simulink model "MPCPF_kinematics"  (R2016a)
settings: Solver=ode4  StartTime=0.0  StopTime=300  FixedStep=Ts  RelTol=1e-3
values from neighbouring files (symbols this model uses):
  Ts = 0.1    [CPFMPC_Lyapunovbased.mat]    (also in CPFMPC_NoTerminalConstraint.mat; Coordination.m; Data_StrategyII_No_Constraint.mat; Data_StrategyI_Constraint.mat = 0.2)
settings Model: Creator=hung  LastModifiedBy=hung

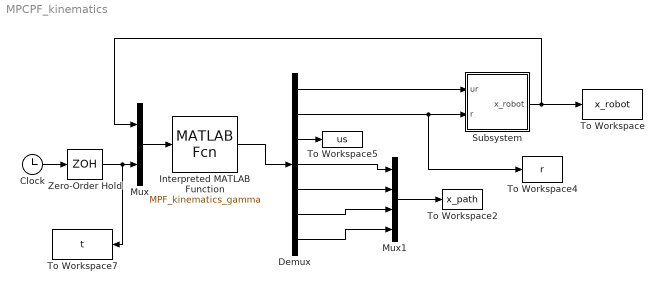
== system MPCPF_kinematics ==
  Clock : Clock
  Demux : Demux  Outputs=7
  Interpreted MATLAB Function : MATLABFcn  MATLABFcn=MPF_kinematics_gamma  OutputDimensions=7
  Mux : Mux  Inputs=2
  Mux1 : Mux
  Subsystem : Subsystem
  To Workspace : ToWorkspace  VariableName=x_robot  SampleTime=-1
  To Workspace2 : ToWorkspace  VariableName=x_path  SampleTime=-1
  To Workspace4 : ToWorkspace  VariableName=r  SampleTime=-1
  To Workspace5 : ToWorkspace  VariableName=us  SampleTime=-1
  To Workspace7 : ToWorkspace  VariableName=t  SampleTime=Ts
  Zero-Order Hold : ZeroOrderHold  SampleTime=Ts
  wires:
  Interpreted MATLAB Function/1 -> Demux/1
  Mux/1 -> Interpreted MATLAB Function/1
  Clock/1 -> Zero-Order Hold/1
  Zero-Order Hold/1 -> Mux/2, To Workspace7/1
  Demux/2 -> To Workspace4/1, Subsystem/2(r)
  Demux/4 -> Mux1/1
  Demux/5 -> Mux1/2
  Mux1/1 -> To Workspace2/1
  Demux/3 -> To Workspace5/1
  Demux/6 -> Mux1/3
  Demux/7 -> Mux1/4
  Demux/1 -> Subsystem/1(ur)
  Subsystem/1(x_robot) -> Mux/1, To Workspace/1

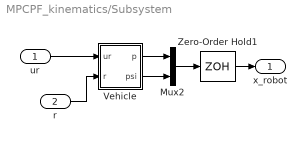
== system MPCPF_kinematics/Subsystem ==
  ur : Inport
  r : Inport  Port=2
  Mux2 : Mux  Inputs=2
  Vehicle : Subsystem
  Zero-Order Hold1 : ZeroOrderHold  SampleTime=Ts
  x_robot : Outport
  wires:
  Vehicle/2(psi) -> Mux2/2
  Mux2/1 -> Zero-Order Hold1/1
  r/1 -> Vehicle/2(r)
  Zero-Order Hold1/1 -> x_robot/1
  Vehicle/1(p) -> Mux2/1
  ur/1 -> Vehicle/1(ur)

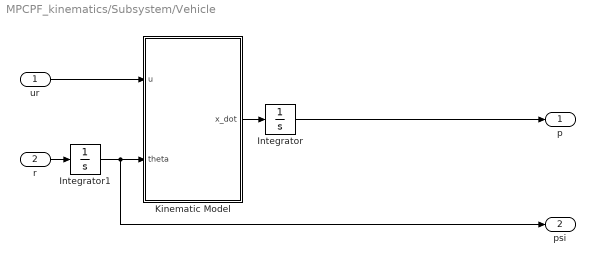
== system MPCPF_kinematics/Subsystem/Vehicle ==
  ur : Inport
  r : Inport  Port=2
  Integrator : Integrator  InitialCondition=[3;0]
  Integrator1 : Integrator
  Kinematic Model : MATLAB Function  TreatAsAtomicUnit=on
  p : Outport
  psi : Outport  Port=2
  wires:
  r/1 -> Integrator1/1
  ur/1 -> Kinematic Model/1(u)
  Kinematic Model/1(x_dot) -> Integrator/1
  Integrator/1 -> p/1
  Integrator1/1 -> psi/1, Kinematic Model/2(theta)

== matlab function MPCPF_kinematics/Subsystem/Vehicle/Kinematic Model ==
  data: u input; x_dot output; theta input
function x_dot = fcn(u,theta)

%% Differential Equation

x_dot=[u*cos(theta); u*sin(theta)];
